simulink model "CS_Cr_simulado_v75R2010a"  (Simulink 7.5)
settings: Solver=ode5  StartTime=0.0  StopTime=10  FixedStep=0.5  RelTol=1e-3
undefined symbols (not defined in the file): A, B
libraries: simulink x2
settings Model: Creator=Equipo-Servo  LastModifiedBy=Servo  ExtModeTrigDuration=10000
settings OptimizationCC: ExpressionDepthLimit=128
settings DebuggingCC: FcnCallInpInsideContextMsg=Enable All
settings HardwareCC: ProdIntDivRoundTo=Zero  ProdEndianess=LittleEndian  ProdHWDeviceType=Generic->32-bit x86 compatible
settings RTWCC: SystemTargetFile=rtwin.tlc  TemplateMakefile=rtwin.tmf  Description=Real-Time Windows Target  ProcessScript=rtwin_make_rtw_hook  RTWCompilerOptimization=On
settings CodeAppCC: MaxIdLength=95  CustomSymbolStrType=$N$R$M_T
settings RTWinTargetCC: TargetLibSuffix=_rtwin.lib  TargetPreCompLibLocation=C:\Program Files\MATLAB\R2014b\toolbox\rtw\targets\rtwin\lib\win64  TargetFunctionLibrary=C89/C90 (ANSI)  MatFileLogging=on

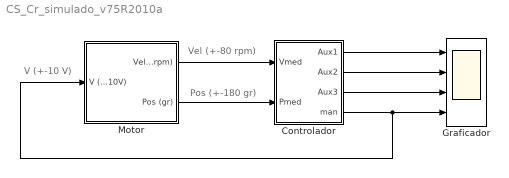
== system CS_Cr_simulado_v75R2010a ==
  note: Vel (+-80 rpm)
  note: Pos (+-180 gr)
  note: V (+-10 V)
  Controlador : Subsystem
  Graficador : Scope  NumInputPorts=4
      settings: TimeRange=10  YMin=-50~-5~-5~-0.5  YMax=50~10~10~1
  Motor : Subsystem
  wires:
  Controlador/4(man) -> Motor/1(V (+-10V)), Graficador/4
  Motor/1(Vel (rpm)) -> Controlador/1(Vmed)
  Motor/2(Pos (gr)) -> Controlador/2(Pmed)
  Controlador/1(Aux1) -> Graficador/1
  Controlador/3(Aux3) -> Graficador/3
  Controlador/2(Aux2) -> Graficador/2

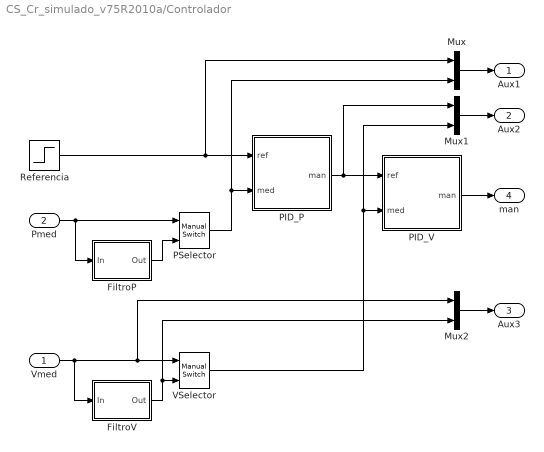
== system CS_Cr_simulado_v75R2010a/Controlador ==
  Vmed : Inport
  Pmed : Inport  Port=2
  FiltroP : Subsystem  mask{N=2, Fc=0.5, Fm=1/0.5}
      mask prompts: N "Orden del filtro (Butterworth)"; Fc "Frecuencia de corte (Fc<Fm/2)"; Fm "Frecuencia de muestreo"
      mask init:
      | Fn = Fm/2;   % Frecuencia de Nyquist
      | [B,A] = butter(N,Fc/Fn);
  FiltroV : Subsystem  mask{N=2, Fc=0.5, Fm=1/0.5}
      mask prompts: N "Orden del filtro (Butterworth)"; Fc "Frecuencia de corte (Fc<Fm/2)"; Fm "Frecuencia de muestreo"
      mask init:
      | Fn = Fm/2;   % Frecuencia de Nyquist
      | [B,A] = butter(N,Fc/Fn);
  Mux : Mux  Inputs=2
  Mux1 : Mux  Inputs=2
  Mux2 : Mux  Inputs=2
  PID_P : Subsystem  mask{P=0.1, I=0, D=0, Tm=0.5, Kb=0, Fc=0.5, Mmx=80, Mmn=-80}
      mask prompts: P "Ganancia Proporcional"; I "Ganancia Integral"; D "Ganancia Derivativa"; Tm "Período de muestreo"; Kb "Ganancia Antiwindup"; Fc "Fc Filtro D"; Mmx "Mando máximo"; Mmn "Mando mínimo"
      mask init:
      | N=2*pi*Fc;
  PID_V : Subsystem  mask{P=0.1, I=0, D=0, Tm=0.5, Kb=0, Fc=0.5, Mmx=10, Mmn=-10}
      mask prompts: P "Ganancia Proporcional"; I "Ganancia Integral"; D "Ganancia Derivativa"; Tm "Período de muestreo"; Kb "Ganancia Antiwindup"; Fc "Fc Filtro D"; Mmx "Mando máximo"; Mmn "Mando mínimo"
      mask init:
      | N=2*pi*Fc;
  PSelector : simulink/Signal Routing/Manual Switch  sw=1  action=0  varsize=off
  Referencia : Step  Time=5  Before=-50  After=50  SampleTime=0
  VSelector : simulink/Signal Routing/Manual Switch  sw=1  action=0  varsize=off
  Aux1 : Outport
  Aux2 : Outport  Port=2
  Aux3 : Outport  Port=3
  man : Outport  Port=4
  wires:
  Referencia/1 -> Mux/1, PID_P/1(ref)
  Pmed/1 -> FiltroP/1(In), PSelector/1
  PID_P/1(man) -> PID_V/1(ref), Mux1/1
  Vmed/1 -> FiltroV/1(In), Mux2/1, VSelector/1
  FiltroV/1(Out) -> Mux2/2, VSelector/2
  VSelector/1 -> PID_V/2(med), Mux1/2
  FiltroP/1(Out) -> PSelector/2
  PSelector/1 -> PID_P/2(med), Mux/2
  Mux/1 -> Aux1/1
  Mux1/1 -> Aux2/1
  Mux2/1 -> Aux3/1
  PID_V/1(man) -> man/1

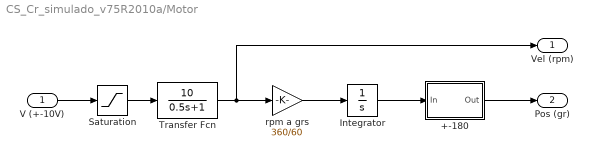
== system CS_Cr_simulado_v75R2010a/Motor ==
  V (+-10V) : Inport
  +-180 : Subsystem
  Integrator : Integrator  InitialCondition=180  UpperSaturationLimit=180  LowerSaturationLimit=-180
  Saturation : Saturate  UpperLimit=10  LowerLimit=-10
  Transfer Fcn : TransferFcn  Numerator=[10]  Denominator=[0.5 1]
  rpm a grs : Gain  Gain=360/60
  Vel (rpm) : Outport
  Pos (gr) : Outport  Port=2
  wires:
  V (+-10V)/1 -> Saturation/1
  Transfer Fcn/1 -> Vel (rpm)/1, rpm a grs/1
  Integrator/1 -> +-180/1(In)
  Saturation/1 -> Transfer Fcn/1
  +-180/1(Out) -> Pos (gr)/1
  rpm a grs/1 -> Integrator/1

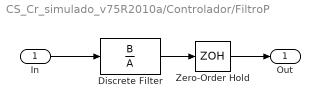
== system CS_Cr_simulado_v75R2010a/Controlador/FiltroP ==
  In : Inport
  Discrete Filter : DiscreteFilter  Numerator=B  Denominator=A  SampleTime=1/Fm
  Zero-Order Hold : ZeroOrderHold  SampleTime=1/Fm
  Out : Outport
  wires:
  Discrete Filter/1 -> Zero-Order Hold/1
  In/1 -> Discrete Filter/1
  Zero-Order Hold/1 -> Out/1

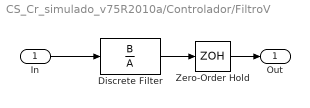
== system CS_Cr_simulado_v75R2010a/Controlador/FiltroV ==
  In : Inport
  Discrete Filter : DiscreteFilter  Numerator=B  Denominator=A  SampleTime=1/Fm
  Zero-Order Hold : ZeroOrderHold  SampleTime=1/Fm
  Out : Outport
  wires:
  In/1 -> Discrete Filter/1
  Discrete Filter/1 -> Zero-Order Hold/1
  Zero-Order Hold/1 -> Out/1

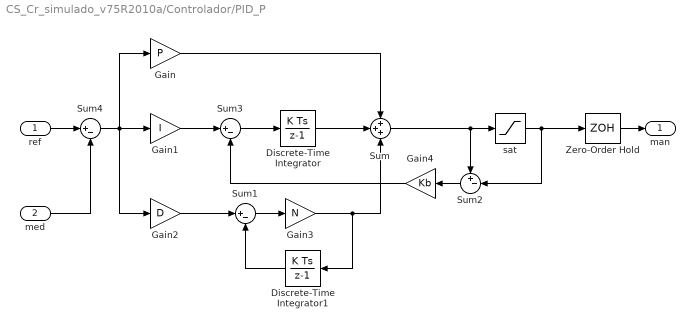
== system CS_Cr_simulado_v75R2010a/Controlador/PID_P ==
  ref : Inport
  med : Inport  Port=2
  Discrete-Time Integrator : DiscreteIntegrator  SampleTime=Tm
  Discrete-Time Integrator1 : DiscreteIntegrator  SampleTime=Tm
  Gain : Gain  Gain=P
  Gain1 : Gain  Gain=I
  Gain2 : Gain  Gain=D
  Gain3 : Gain  Gain=N
  Gain4 : Gain  Gain=Kb
  Sum : Sum  Inputs=+++
  Sum1 : Sum  Inputs=|+-
  Sum2 : Sum  Inputs=+-|
  Sum3 : Sum  Inputs=|+-
  Sum4 : Sum  Inputs=|+-
  Zero-Order Hold : ZeroOrderHold  SampleTime=Tm
  sat : Saturate  UpperLimit=Mmx  LowerLimit=Mmn
  man : Outport
  wires:
  Gain2/1 -> Sum1/1
  Discrete-Time Integrator1/1 -> Sum1/2
  Sum3/1 -> Discrete-Time Integrator/1
  Sum4/1 -> Gain2/1, Gain/1, Gain1/1
  Gain3/1 -> Sum/3, Discrete-Time Integrator1/1
  Gain/1 -> Sum/1
  Gain4/1 -> Sum3/2
  Sum1/1 -> Gain3/1
  Discrete-Time Integrator/1 -> Sum/2
  Sum2/1 -> Gain4/1
  Sum/1 -> Sum2/1, sat/1
  sat/1 -> Sum2/2, Zero-Order Hold/1
  Gain1/1 -> Sum3/1
  med/1 -> Sum4/2
  ref/1 -> Sum4/1
  Zero-Order Hold/1 -> man/1

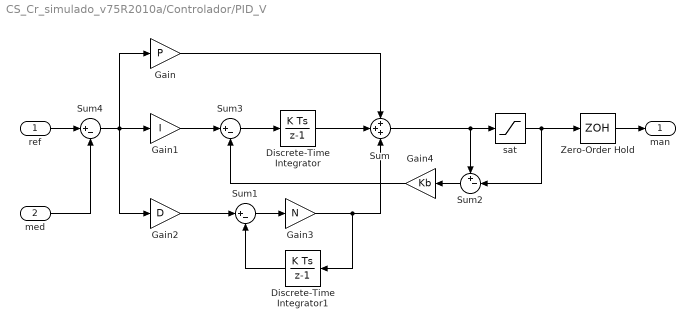
== system CS_Cr_simulado_v75R2010a/Controlador/PID_V ==
  ref : Inport
  med : Inport  Port=2
  Discrete-Time Integrator : DiscreteIntegrator  SampleTime=Tm
  Discrete-Time Integrator1 : DiscreteIntegrator  SampleTime=Tm
  Gain : Gain  Gain=P
  Gain1 : Gain  Gain=I
  Gain2 : Gain  Gain=D
  Gain3 : Gain  Gain=N
  Gain4 : Gain  Gain=Kb
  Sum : Sum  Inputs=+++
  Sum1 : Sum  Inputs=|+-
  Sum2 : Sum  Inputs=+-|
  Sum3 : Sum  Inputs=|+-
  Sum4 : Sum  Inputs=|+-
  Zero-Order Hold : ZeroOrderHold  SampleTime=Tm
  sat : Saturate  UpperLimit=Mmx  LowerLimit=Mmn
  man : Outport
  wires:
  ref/1 -> Sum4/1
  med/1 -> Sum4/2
  Gain1/1 -> Sum3/1
  sat/1 -> Zero-Order Hold/1, Sum2/2
  Sum/1 -> sat/1, Sum2/1
  Sum2/1 -> Gain4/1
  Discrete-Time Integrator/1 -> Sum/2
  Sum1/1 -> Gain3/1
  Gain4/1 -> Sum3/2
  Gain/1 -> Sum/1
  Gain3/1 -> Discrete-Time Integrator1/1, Sum/3
  Sum4/1 -> Gain1/1, Gain/1, Gain2/1
  Sum3/1 -> Discrete-Time Integrator/1
  Discrete-Time Integrator1/1 -> Sum1/2
  Gain2/1 -> Sum1/1
  Zero-Order Hold/1 -> man/1

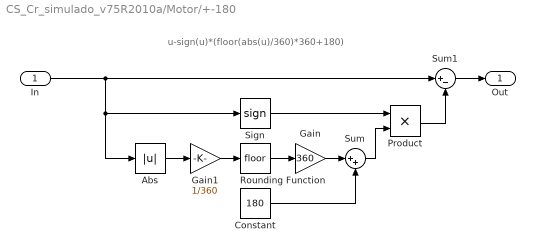
== system CS_Cr_simulado_v75R2010a/Motor/+-180 ==
  note: u-sign(u)*(floor(abs(u)/360)*360+180)
  In : Inport
  Abs : Abs
  Constant : Constant  Value=180
  Gain : Gain  Gain=360
  Gain1 : Gain  Gain=1/360
  Product : Product
  Rounding Function : Rounding
  Sign : Signum
  Sum : Sum  Inputs=|++
  Sum1 : Sum  Inputs=|+-
  Out : Outport
  wires:
  Sum/1 -> Product/2
  Constant/1 -> Sum/2
  Sign/1 -> Product/1
  Gain1/1 -> Rounding Function/1
  Gain/1 -> Sum/1
  Rounding Function/1 -> Gain/1
  Sum1/1 -> Out/1
  Abs/1 -> Gain1/1
  Product/1 -> Sum1/2
  In/1 -> Abs/1, Sign/1, Sum1/1
